simulink model "MSBR_nn_PID_Thot"  (R2016b)
settings: Solver=VariableStepAuto  StartTime=0.0  StopTime=simtime  RelTol=1e-3
values from neighbouring files (symbols this model uses):
  a_b = 1.656E-05    (= 1.656e-05)    [Parameters_new_nodal.m]
  A_Bgn = A_Bg/nn_Bg    [Parameters_new_nodal.m]
  a_f = -8.172E-05    (= -8.172e-05)    [Parameters_new_nodal.m]
  A_fgboren = A_fgbore/nn_fdn    (= 52.5696341877)    [Parameters_new_nodal.m]
  A_fgsleidn = A_fgsleid/nn_fup    (= 29.0039361035)    [Parameters_new_nodal.m]
  A_fgsleodn = A_fgsleod/nn_fdn    (= 43.5059041553)    [Parameters_new_nodal.m]
  a_g = 2.016E-05    (= 2.016e-05)    [Parameters_new_nodal.m]
  A_ggin = A_ggi/nn_gg    [Parameters_new_nodal.m]
  A_ggon = A_ggo/nn_gg    [Parameters_new_nodal.m]
  beta = [2.290E-04, 8.320E-04, 7.100E-04, 8.520E-04, 1.710E-04, 1.020E-04]    [Parameters_new_nodal.m]
  beta_t = sum(beta)    [Parameters_new_nodal.m]
  Cp_B = 9.211E-04    (= 0.0009211)    [Parameters_new_nodal.m]
  Cp_f = 2.302E-03    (= 0.002302)    [Parameters_new_nodal.m]
  Cp_g = 1.679E-03    (= 0.001679)    [Parameters_new_nodal.m]
  h_Bg = 2.839E-03    (= 0.002839)    [Parameters_new_nodal.m]
  h_fgi = 9.176E-03    (= 0.009176)    [Parameters_new_nodal.m]
  h_fgo = 8.165E-03    (= 0.008165)    [Parameters_new_nodal.m]
  h_ggi = cond_g/l_i    [Parameters_new_nodal.m]
  h_ggo = cond_g/l_o    [Parameters_new_nodal.m]
  hA_p1 = h_p*A_phe/4    (= 2.993352)    [Parameters_new_nodal.m]
  hA_p2 = h_p*A_phe/4    (= 2.993352)    [Parameters_new_nodal.m]
  hA_p3 = h_p*A_phe/4    (= 2.993352)    [Parameters_new_nodal.m]
  hA_p4 = h_p*A_phe/4    (= 2.993352)    [Parameters_new_nodal.m]
  hA_pb1 = 7.150E-01    (= 0.715)    [Parameters_new_nodal.m]
  hA_pb2 = 7.150E-01    (= 0.715)    [Parameters_new_nodal.m]
  hA_s1 = h_s*A_phe/4    (= 5.85606)    [Parameters_new_nodal.m]
  hA_s2 = h_s*A_phe/4    (= 5.85606)    [Parameters_new_nodal.m]
  hA_s3 = h_s*A_phe/4    (= 5.85606)    [Parameters_new_nodal.m]
  hA_s4 = h_s*A_phe/4    (= 5.85606)    [Parameters_new_nodal.m]
  hA_s5 = 7.150E-01    (= 0.715)    [Parameters_new_nodal.m]
  hA_s6 = 7.150E-01    (= 0.715)    [Parameters_new_nodal.m]
  k_Ba1 = 8.500E-03/2    (= 0.00425)    [Parameters_new_nodal.m]
  k_Ba2 = 8.500E-03/2    (= 0.00425)    [Parameters_new_nodal.m]
  k_Bb1 = 8.500E-03/2    (= 0.00425)    [Parameters_new_nodal.m]
  k_Bb2 = 8.500E-03/2    (= 0.00425)    [Parameters_new_nodal.m]
  k_BL = 1-k_core    [Parameters_new_nodal.m]
  k_f1a1 = 2.210E-01/2    (= 0.1105)    [Parameters_new_nodal.m]
  k_f1a2 = 2.210E-01/2    (= 0.1105)    [Parameters_new_nodal.m]
  k_f1b1 = 2.210E-01/2    (= 0.1105)    [Parameters_new_nodal.m]
  k_f1b2 = 2.210E-01/2    (= 0.1105)    [Parameters_new_nodal.m]
  k_f2a1 = 2.210E-01/2    (= 0.1105)    [Parameters_new_nodal.m]
  k_f2a2 = 2.210E-01/2    (= 0.1105)    [Parameters_new_nodal.m]
  k_f2b1 = 2.210E-01/2    (= 0.1105)    [Parameters_new_nodal.m]
  k_f2b2 = 2.210E-01/2    (= 0.1105)    [Parameters_new_nodal.m]
  k_g1a = rkmf*m_g1a    [Parameters_new_nodal.m]
  k_g1b = rkmf*m_g1b    [Parameters_new_nodal.m]
  k_g2a = rkmf*m_g2a    [Parameters_new_nodal.m]
  k_g2b = rkmf*m_g2b    [Parameters_new_nodal.m]
  k_g3a = rkmf*m_g3a    [Parameters_new_nodal.m]
  k_g3b = rkmf*m_g3b    [Parameters_new_nodal.m]
  k_g4a = (rkmB*m_gB+rkmf*(m_g4a+m_g4b-m_gB))/2    [Parameters_new_nodal.m]
  k_g4b = (rkmB*m_gB+rkmf*(m_g4a+m_g4b-m_gB))/2    [Parameters_new_nodal.m]
  Lam = 3.300E-04    (= 0.00033)    [Parameters_new_nodal.m]
  lam = [1.260E-02, 3.370E-02, 1.390E-01, 3.250E-01, 1.130E+00, 2.500E+00]    [Parameters_new_nodal.m]
  m_Ba1 = m_B/nn_B    (= 2092.75)    [Parameters_new_nodal.m]
  m_Ba2 = m_B/nn_B    (= 2092.75)    [Parameters_new_nodal.m]
  m_Bb1 = m_B/nn_B    (= 2092.75)    [Parameters_new_nodal.m]
  m_Bb2 = m_B/nn_B    (= 2092.75)    [Parameters_new_nodal.m]
  m_BL = 22804.35    [Parameters_new_nodal.m]
  m_Bm = W_B    (= 271.65)    [Parameters_new_nodal.m]
  m_f1a1 = mn_f    (= 1004.5)    [Parameters_new_nodal.m]
  m_f1a2 = mn_f    (= 1004.5)    [Parameters_new_nodal.m]
  m_f1b1 = mn_f    (= 1004.5)    [Parameters_new_nodal.m]
  m_f1b2 = mn_f    (= 1004.5)    [Parameters_new_nodal.m]
  m_f2a1 = mn_f    (= 1004.5)    [Parameters_new_nodal.m]
  m_f2a2 = mn_f    (= 1004.5)    [Parameters_new_nodal.m]
  m_f2b1 = mn_f    (= 1004.5)    [Parameters_new_nodal.m]
  m_f2b2 = mn_f    (= 1004.5)    [Parameters_new_nodal.m]
  m_g1a = (rho_g*(pi*r_msle^2 - pi*(sle_ID/2)^2)*l_cell*n_cell/2)    [Parameters_new_nodal.m]
  m_g1b = (rho_g*(pi*r_msle^2 - pi*(sle_ID/2)^2)*l_cell*n_cell/2)    [Parameters_new_nodal.m]
  m_g2a = (rho_g*(pi*(sle_OD/2)^2 - pi*r_msle^2)*l_cell*n_cell/2)    [Parameters_new_nodal.m]
  m_g2b = (rho_g*(pi*(sle_OD/2)^2 - pi*r_msle^2)*l_cell*n_cell/2)    [Parameters_new_nodal.m]
  m_g3a = (rho_g*(pi*r_mhex^2 - pi*(bore_OD/2)^2)*l_cell*n_cell/2)    [Parameters_new_nodal.m]
  m_g3b = (rho_g*(pi*r_mhex^2 - pi*(bore_OD/2)^2)*l_cell*n_cell/2)    [Parameters_new_nodal.m]
  m_g4a = (rho_g*(A_hex - pi*r_mhex^2)*l_cell*n_cell/2)    [Parameters_new_nodal.m]
  m_g4b = (rho_g*(A_hex - pi*r_mhex^2)*l_cell*n_cell/2)    [Parameters_new_nodal.m]
  m_pb1 = mcp_pb1/Cp_B    (= 430.680707849)    [Parameters_new_nodal.m]
  m_pb2 = mcp_pb2/Cp_B    (= 430.680707849)    [Parameters_new_nodal.m]
  m_s5 = mcp_s5/Cp_s    (= 1575.26254376)    [Parameters_new_nodal.m]
  m_s6 = mcp_s6/Cp_s    (= 1575.26254376)    [Parameters_new_nodal.m]
  m_sb = 4808    [Parameters_new_nodal.m]
  m_sr = 3062    [Parameters_new_nodal.m]
  mb_cpb = 3.297E+01    (= 32.97)    [Parameters_new_nodal.m]
  mcp_p1 = mn_p*Cp_p    (= 5.3043835)    [Parameters_new_nodal.m]
  mcp_p2 = mn_p*Cp_p    (= 5.3043835)    [Parameters_new_nodal.m]
  mcp_p3 = mn_p*Cp_p    (= 5.3043835)    [Parameters_new_nodal.m]
  mcp_p4 = mn_p*Cp_p    (= 5.3043835)    [Parameters_new_nodal.m]
  mcp_pb1 = 3.967E-01    (= 0.3967)    [Parameters_new_nodal.m]
  mcp_pb2 = 3.967E-01    (= 0.3967)    [Parameters_new_nodal.m]
  mcp_s1 = mn_s*Cp_s    (= 6.80458)    [Parameters_new_nodal.m]
  mcp_s2 = mn_s*Cp_s    (= 6.80458)    [Parameters_new_nodal.m]
  mcp_s3 = mn_s*Cp_s    (= 6.80458)    [Parameters_new_nodal.m]
  mcp_s4 = mn_s*Cp_s    (= 6.80458)    [Parameters_new_nodal.m]
  mcp_s5 = 2.7E+00    (= 2.7)    [Parameters_new_nodal.m]
  mcp_s6 = 2.7E+00    (= 2.7)    [Parameters_new_nodal.m]
  mcp_t1 = 2.158    [Parameters_new_nodal.m]
  mcp_t2 = 2.158    [Parameters_new_nodal.m]
  mcp_t3 = m_t*cp_t    (= 0.51412242)    [Parameters_new_nodal.m]
  mn_m = W_f    (= 1373)    [Parameters_new_nodal.m]
  mn_ms = mn_m    (= 1373)    [Parameters_new_nodal.m]
  mn_p = m_p/nn_p    (= 2304.25)    [Parameters_new_nodal.m]
  mn_s = m_s/nn_s    (= 3970)    [Parameters_new_nodal.m]
  mr_cpr = 1.050E+01    (= 10.5)    [Parameters_new_nodal.m]
  n_frac0 = 1    [Parameters_new_nodal.m]
  P = 556.0    (= 556)    [Parameters_new_nodal.m]
  p_b = 0.87*P    (= 483.72)    [Parameters_new_nodal.m]
  p_r = 0.13*P    (= 72.28)    [Parameters_new_nodal.m]
  T0_b2 = 676.66    [Parameters_new_nodal.m]
  T0_Ba1 = T0_b2-(T0_b2-T_b_in)*(1/4)    (= 662.7725)    [Parameters_new_nodal.m]
  T0_Ba2 = T0_b2    (= 676.66)    [Parameters_new_nodal.m]
  T0_Bb1 = T0_b2-(T0_b2-T_b_in)*(3/4)    (= 634.9975)    [Parameters_new_nodal.m]
  T0_Bb2 = T0_b2-(T0_b2-T_b_in)*(2/4)    (= 648.885)    [Parameters_new_nodal.m]
  T0_BL = T0_Ba2    (= 676.66)    [Parameters_new_nodal.m]
  T0_Bm = T0_Ba2    (= 676.66)    [Parameters_new_nodal.m]
  T0_f1a1 = T0_f4-(T0_f4-Tf_in)*(2/8)    (= 662.7725)    [Parameters_new_nodal.m]
  T0_f1a2 = T0_f4-(T0_f4-Tf_in)*(3/8)    (= 641.93875)    [Parameters_new_nodal.m]
  T0_f1b1 = T0_f4    (= 704.44)    [Parameters_new_nodal.m]
  T0_f1b2 = T0_f4-(T0_f4-Tf_in)*(1/8)    (= 683.60625)    [Parameters_new_nodal.m]
  T0_f2a1 = T0_f4-(T0_f4-Tf_in)*(4/8)    (= 621.105)    [Parameters_new_nodal.m]
  T0_f2a2 = T0_f4-(T0_f4-Tf_in)*(5/8)    (= 600.27125)    [Parameters_new_nodal.m]
  ... (+47 more)
undefined symbols (not defined in the file or in its folder): C0
libraries: simulink x3
settings Model: Creator=VIKRAM SINGH  LastModifiedBy=matthew

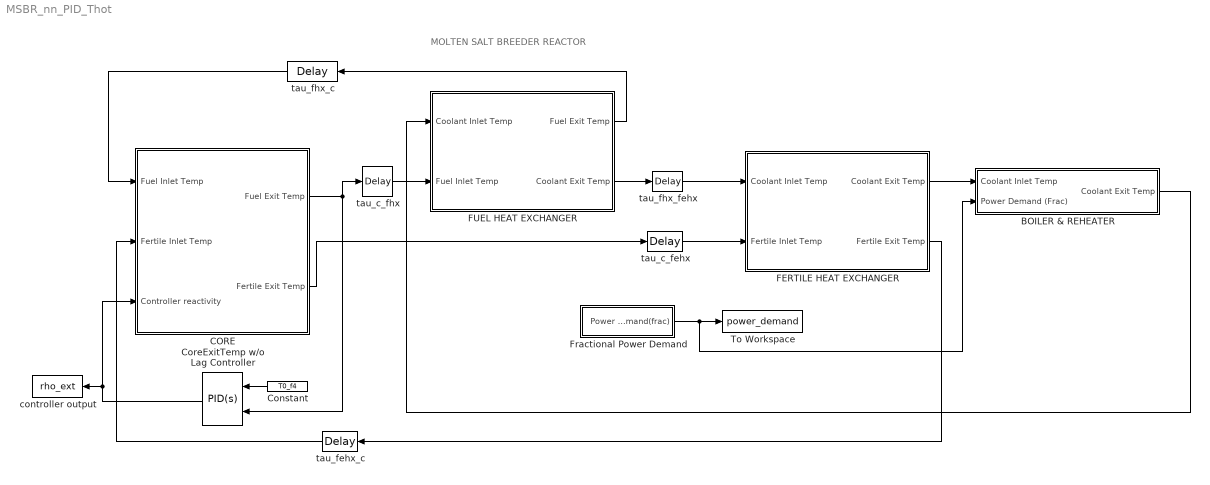
== system MSBR_nn_PID_Thot ==
  note: MOLTEN SALT BREEDER REACTOR
  BOILER & REHEATER : Subsystem
  CORE : Subsystem
  Constant : Constant  Value=T0_f4
  CoreExitTemp w/o Lag Controller : simulink/Continuous/PID Controller (2DOF)  Controller=PID  TimeDomain=Continuous-time  SampleTime=-1  IntegratorMethod=Forward Euler  FilterMethod=Forward Euler  Form=Parallel  UseFilter=on  ControllerParametersSource=internal  P=6.0515509831089e-05  I=4.82645542777223e-05  D=0  N=100  b=1  c=1  InitialConditionSource=internal  InitialConditionForIntegrator=0  InitialConditionForFilter=0  ExternalReset=none  LimitOutput=off  UpperSaturationLimit=inf  LowerSaturationLimit=-inf  LinearizeAsGain=on  AntiWindupMode=none  Kb=1  TrackingMode=off  Kt=1  PParamMin=[]  PParamMax=[]  IParamMin=[]  IParamMax=[]  DParamMin=[]  DParamMax=[]  NParamMin=[]  NParamMax=[]  bParamMin=[]  bParamMax=[]  cParamMin=[]  cParamMax=[]  KbParamMin=[]  KbParamMax=[]  KtParamMin=[]  KtParamMax=[]  POutMin=[]  POutMax=[]  IOutMin=[]  IOutMax=[]  DOutMin=[]  DOutMax=[]  NOutMin=[]  NOutMax=[]  bOutMin=[]  bOutMax=[]  cOutMin=[]  cOutMax=[]  KbOutMin=[]  KbOutMax=[]  KtOutMin=[]  KtOutMax=[]  IntegratorOutMin=[]  IntegratorOutMax=[]  FilterOutMin=[]  FilterOutMax=[]  SumOutMin=[]  SumOutMax=[]  Sum1OutMin=[]  Sum1OutMax=[]  Sum2OutMin=[]  Sum2OutMax=[]  Sum3OutMin=[]  Sum3OutMax=[]  SumI1OutMin=[]  SumI1OutMax=[]  SumI2OutMin=[]  SumI2OutMax=[]  SumI3OutMin=[]  SumI3OutMax=[]  SumDOutMin=[]  SumDOutMax=[]  SaturationOutMin=[]  SaturationOutMax=[]  IntegratorContinuousStateAttributes=''  IntegratorStateMustResolveToSignalObject=off  IntegratorRTWStateStorageClass=Auto  FilterContinuousStateAttributes=''  FilterStateMustResolveToSignalObject=off  FilterRTWStateStorageClass=Auto  DifferentiatorICPrevScaledInput=0  DifferentiatorOutMin=[]  DifferentiatorOutMax=[]
  FERTILE HEAT EXCHANGER : Subsystem
  FUEL HEAT EXCHANGER : Subsystem
  Fractional Power Demand : Subsystem
  To Workspace : ToWorkspace  VariableName=power_demand  SampleTime=-1
  controller output : ToWorkspace  VariableName=rho_ext  SampleTime=-1
  tau_c_fehx : TransportDelay  DelayTime=tau_c_fehx  InitialOutput=T0_b2  BufferSize=4096
  tau_c_fhx : TransportDelay  DelayTime=tau_c_fhx  InitialOutput=T0_f4  BufferSize=4096
  tau_fehx_c : TransportDelay  DelayTime=tau_fehx_c  InitialOutput=T0_pb2  BufferSize=4096
  tau_fhx_c : TransportDelay  DelayTime=tau_fhx_c  InitialOutput=T0_p4  BufferSize=4096
  tau_fhx_fehx : TransportDelay  DelayTime=tau_fhx_fehx  InitialOutput=T0_s4  BufferSize=4096
  wires:
  FUEL HEAT EXCHANGER/2(Coolant Exit Temp) -> tau_fhx_fehx/1
  FERTILE HEAT EXCHANGER/2(Fertile Exit Temp) -> tau_fehx_c/1
  FERTILE HEAT EXCHANGER/1(Coolant Exit Temp) -> BOILER & REHEATER/1(Coolant Inlet Temp)
  tau_c_fhx/1 -> FUEL HEAT EXCHANGER/2(Fuel Inlet Temp)
  tau_c_fehx/1 -> FERTILE HEAT EXCHANGER/2(Fertile Inlet Temp)
  FUEL HEAT EXCHANGER/1(Fuel Exit Temp) -> tau_fhx_c/1
  tau_fhx_fehx/1 -> FERTILE HEAT EXCHANGER/1(Coolant Inlet Temp)
  BOILER & REHEATER/1(Coolant Exit Temp) -> FUEL HEAT EXCHANGER/1(Coolant Inlet Temp)
  tau_fhx_c/1 -> CORE/1(Fuel Inlet Temp)
  tau_fehx_c/1 -> CORE/2(Fertile Inlet Temp)
  CORE/2(Fertile Exit Temp) -> tau_c_fehx/1
  CoreExitTemp w/o Lag Controller/1 -> CORE/3(Controller reactivity), controller output/1
  Fractional Power Demand/1(Power Demand(frac)) -> BOILER & REHEATER/2(Power Demand (Frac)), To Workspace/1
  Constant/1 -> CoreExitTemp w/o Lag Controller/1
  CORE/1(Fuel Exit Temp) -> CoreExitTemp w/o Lag Controller/2, tau_c_fhx/1

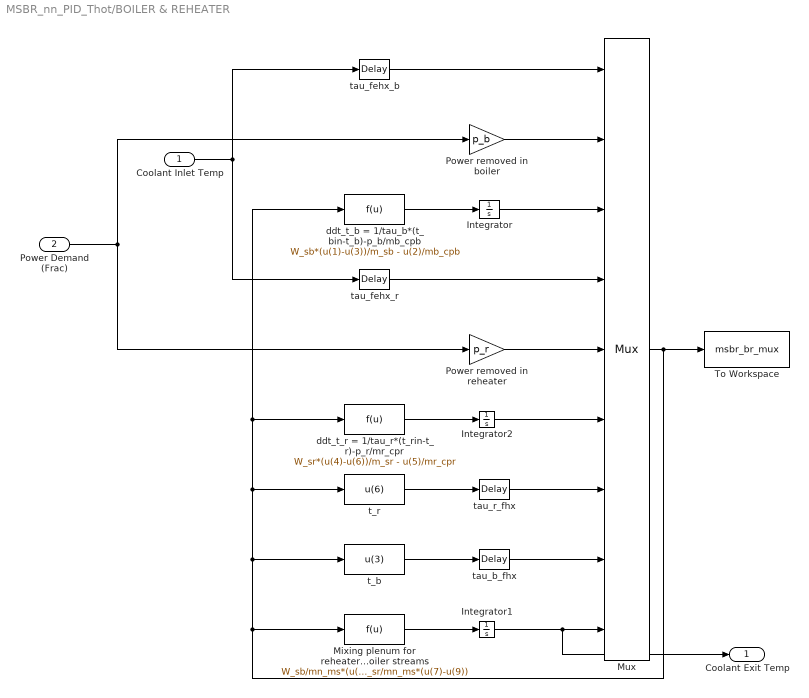
== system MSBR_nn_PID_Thot/BOILER & REHEATER ==
  Coolant Inlet Temp : Inport
  Power Demand (Frac) : Inport  Port=2
  Integrator : Integrator  InitialCondition=Ts_in
  Integrator1 : Integrator  InitialCondition=Ts_in
  Integrator2 : Integrator  InitialCondition=Ts_in
  Mixing plenum for reheater and boiler streams : Fcn  Expr=W_sb/mn_ms*(u(8)-u(9))+W_sr/mn_ms*(u(7)-u(9))
  Mux : Mux  Inputs=9
      settings: DisplayOption=signals
  Power removed in boiler : Gain  Gain=p_b
  Power removed in reheater : Gain  Gain=p_r
  To Workspace : ToWorkspace  VariableName=msbr_br_mux  SampleTime=-1
  ddt_t_b = 1/tau_b*(t_bin-t_b)-p_b/mb_cpb : Fcn  Expr=W_sb*(u(1)-u(3))/m_sb - u(2)/mb_cpb
  ddt_t_r = 1/tau_r*(t_rin-t_r)-p_r/mr_cpr : Fcn  Expr=W_sr*(u(4)-u(6))/m_sr - u(5)/mr_cpr
  t_b : Fcn  Expr=u(3)
  t_r : Fcn  Expr=u(6)
  tau_b_fhx : TransportDelay  DelayTime=tau_b_fhx  InitialOutput=Ts_in  BufferSize=4096
  tau_fehx_b : TransportDelay  DelayTime=tau_fehx_b  InitialOutput=T0_s6  BufferSize=4096
  tau_fehx_r : TransportDelay  DelayTime=tau_fehx_r  InitialOutput=T0_s6  BufferSize=4096
  tau_r_fhx : TransportDelay  DelayTime=tau_r_fhx  InitialOutput=Ts_in  BufferSize=4096
  Coolant Exit Temp : Outport
  wires:
  Coolant Inlet Temp/1 -> tau_fehx_r/1, tau_fehx_b/1
  Power removed in boiler/1 -> Mux/2
  Integrator/1 -> Mux/3
  ddt_t_r = 1/tau_r*(t_rin-t_r)-p_r/mr_cpr/1 -> Integrator2/1
  ddt_t_b = 1/tau_b*(t_bin-t_b)-p_b/mb_cpb/1 -> Integrator/1
  Mux/1 -> t_b/1, t_r/1, ddt_t_r = 1/tau_r*(t_rin-t_r)-p_r/mr_cpr/1, ddt_t_b = 1/tau_b*(t_bin-t_b)-p_b/mb_cpb/1, Mixing plenum for reheater and boiler streams/1, To Workspace/1
  tau_fehx_r/1 -> Mux/4
  Power removed in reheater/1 -> Mux/5
  Integrator2/1 -> Mux/6
  Mixing plenum for reheater and boiler streams/1 -> Integrator1/1
  Integrator1/1 -> Coolant Exit Temp/1, Mux/9
  tau_b_fhx/1 -> Mux/8
  tau_r_fhx/1 -> Mux/7
  t_r/1 -> tau_r_fhx/1
  t_b/1 -> tau_b_fhx/1
  tau_fehx_b/1 -> Mux/1
  Power Demand (Frac)/1 -> Power removed in boiler/1, Power removed in reheater/1

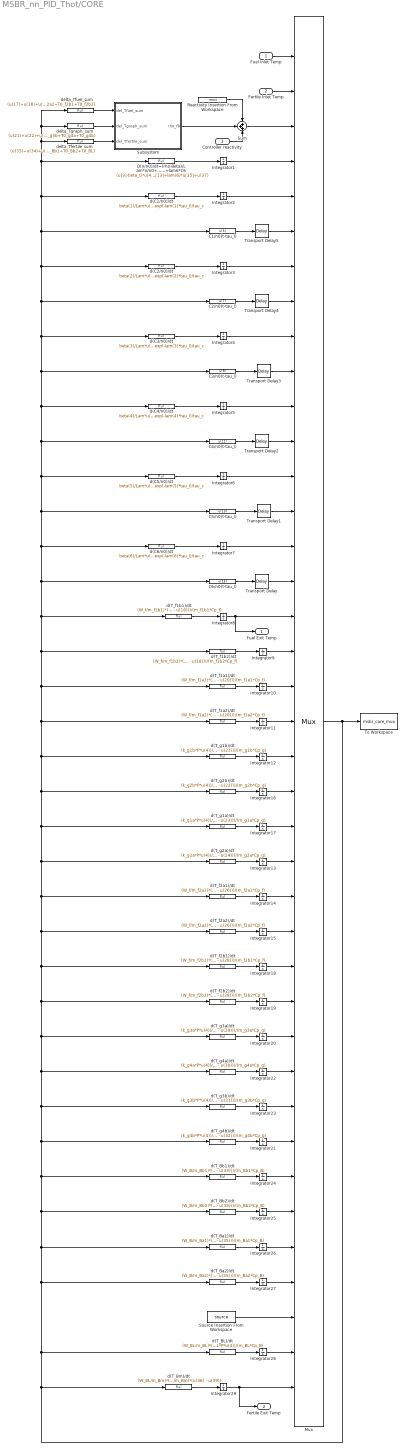
== system MSBR_nn_PID_Thot/CORE ==
  Fuel Inlet Temp : Inport
  Fertile Inlet Temp : Inport  Port=2
  Controller reactivity : Inport  Port=3
  C1/n0(t-tau_l) : Fcn  Expr=u(5)
  C2/n0(t-tau_l) : Fcn  Expr=u(7)
  C3/n0(t-tau_l) : Fcn  Expr=u(9)
  C4/n0(t-tau_l) : Fcn  Expr=u(11)
  C5/n0(t-tau_l) : Fcn  Expr=u(13)
  C6/n0(t-tau_l) : Fcn  Expr=u(15)
  D(n/n0)/dt=(rho-Beta)/Lam*n/n0+lam1*C1+...+lam6*C6 : Fcn  Expr=(u[3]-beta_t)*u[4]/Lam+lam(1)*u[5]+lam(2)*u[7]+lam(3)*u[9]+lam(4)*u[11]+lam(5)*u[13]+lam(6)*u[15]+u(37)
  Integrator1 : Integrator  InitialCondition=n_frac0
  Integrator10 : Integrator  InitialCondition=T0_f1a1
  Integrator11 : Integrator  InitialCondition=T0_f1a2
  Integrator12 : Integrator  InitialCondition=T0_g1b
  Integrator13 : Integrator  InitialCondition=T0_g2a
  Integrator14 : Integrator  InitialCondition=T0_f2a1
  Integrator15 : Integrator  InitialCondition=T0_f2a2
  Integrator16 : Integrator  InitialCondition=T0_g2b
  Integrator17 : Integrator  InitialCondition=T0_g1a
  Integrator18 : Integrator  InitialCondition=T0_f2b1
  Integrator19 : Integrator  InitialCondition=T0_f2b2
  Integrator2 : Integrator  InitialCondition=C0(1)
  Integrator20 : Integrator  InitialCondition=T0_g3a
  Integrator21 : Integrator  InitialCondition=T0_g4b
  Integrator22 : Integrator  InitialCondition=T0_g4a
  Integrator23 : Integrator  InitialCondition=T0_g3b
  Integrator24 : Integrator  InitialCondition=T0_Bb1
  Integrator25 : Integrator  InitialCondition=T0_Bb2
  Integrator26 : Integrator  InitialCondition=T0_Ba1
  Integrator27 : Integrator  InitialCondition=T0_Ba2
  Integrator28 : Integrator  InitialCondition=T0_BL
  Integrator29 : Integrator  InitialCondition=T0_Bm
  Integrator3 : Integrator  InitialCondition=C0(2)
  Integrator4 : Integrator  InitialCondition=C0(3)
  Integrator5 : Integrator  InitialCondition=C0(4)
  Integrator6 : Integrator  InitialCondition=C0(5)
  Integrator7 : Integrator  InitialCondition=C0(6)
  Integrator8 : Integrator  InitialCondition=T0_f1b1
  Integrator9 : Integrator  InitialCondition=T0_f1b2
  Mux : Mux  Inputs=39
      settings: DisplayOption=signals
  Reactivity Insertion From Workspace : FromWorkspace  VariableName=react  SampleTime=1  Interpolate=off  OutputAfterFinalValue=Holding final value
  Source Insertion From Workspace : FromWorkspace  VariableName=source  SampleTime=1  Interpolate=off  OutputAfterFinalValue=Holding final value
  Subsystem : Subsystem
  Sum : Sum  Inputs=+++
  To Workspace : ToWorkspace  VariableName=msbr_core_mux  SampleTime=-1
  Transport Delay : TransportDelay  DelayTime=tau_l  InitialOutput=C0(6)  BufferSize=4096
  Transport Delay1 : TransportDelay  DelayTime=tau_l  InitialOutput=C0(5)  BufferSize=4096
  Transport Delay2 : TransportDelay  DelayTime=tau_l  InitialOutput=C0(4)  BufferSize=4096
  Transport Delay3 : TransportDelay  DelayTime=tau_l  InitialOutput=C0(3)  BufferSize=4096
  Transport Delay4 : TransportDelay  DelayTime=tau_l  InitialOutput=C0(2)  BufferSize=4096
  Transport Delay5 : TransportDelay  DelayTime=tau_l  InitialOutput=C0(1)  BufferSize=4096
  d(C1/n0)/dt : Fcn  Expr=beta(1)/Lam*u(4)-lam(1)*u(5)-u(5)/tau_c+u(6)*exp(-lam(1)*tau_l)/tau_c
  d(C2/n0)/dt : Fcn  Expr=beta(2)/Lam*u(4)-lam(2)*u(7)-u(7)/tau_c+u(8)*exp(-lam(2)*tau_l)/tau_c
  d(C3/n0)/dt : Fcn  Expr=beta(3)/Lam*u(4)-lam(3)*u(9)-u(9)/tau_c+u(10)*exp(-lam(3)*tau_l)/tau_c
  d(C4/n0)/dt : Fcn  Expr=beta(4)/Lam*u(4)-lam(4)*u(11)-u(11)/tau_c+u(12)*exp(-lam(4)*tau_l)/tau_c
  d(C5/n0)/dt : Fcn  Expr=beta(5)/Lam*u(4)-lam(5)*u(13)-u(13)/tau_c+u(14)*exp(-lam(5)*tau_l)/tau_c
  d(C6/n0)/dt : Fcn  Expr=beta(6)/Lam*u(4)-lam(6)*u(15)-u(15)/tau_c+u(16)*exp(-lam(6)*tau_l)/tau_c
  d(T_BL)/dt : Fcn  Expr=(W_BL/m_BL)*(u(2) - u(38)) + (k_BL*P*u(4))/(m_BL*Cp_B)
  d(T_Ba1)/dt : Fcn  Expr=(W_B/m_Ba1)*(u(34) - u(35)) + (k_Ba1*P*u(4))/(m_Ba1*Cp_B) + (h_Bg*A_Bgn*(u(30) - u(35)))/(m_Ba1*Cp_B)
  d(T_Ba2)/dt : Fcn  Expr=(W_B/m_Ba2)*(u(35) - u(36)) + (k_Ba2*P*u(4))/(m_Ba2*Cp_B) + (h_Bg*A_Bgn*(u(30) - u(35)))/(m_Ba2*Cp_B)
  d(T_Bb1)/dt : Fcn  Expr=(W_B/m_Bb1)*(u(2) - u(33)) + (k_Bb1*P*u(4))/(m_Bb1*Cp_B) + (h_Bg*A_Bgn*(u(32) - u(33)))/(m_Bb1*Cp_B)
  d(T_Bb2)/dt : Fcn  Expr=(W_B/m_Bb2)*(u(33) - u(34)) + (k_Bb2*P*u(4))/(m_Bb2*Cp_B) + (h_Bg*A_Bgn*(u(32) - u(33)))/(m_Bb2*Cp_B)
  d(T_Bm)/dt : Fcn  Expr=(W_BL/m_Bm)*(u(38) - u(39)) + (W_B/m_Bm)*(u(36) - u(39))
  d(T_f1a1)/dt : Fcn  Expr=(W_f/m_f1a1)*(u(20) - u(19)) + (k_f1a1*P*u(4))/(m_f1a1*Cp_f) + (h_fgi*A_fgsleidn*(u(23) - u(20)))/(m_f1a1*Cp_f)
  d(T_f1a2)/dt : Fcn  Expr=(W_f/m_f1a2)*(u(25) - u(20)) + (k_f1a2*P*u(4))/(m_f1a2*Cp_f) + (h_fgi*A_fgsleidn*(u(23) - u(20)))/(m_f1a2*Cp_f)
  d(T_f1b1)/dt : Fcn  Expr=(W_f/m_f1b1)*(u(18) - u(17)) + (k_f1b1*P*u(4))/(m_f1b1*Cp_f) + (h_fgi*A_fgsleidn*(u(21) - u(18)))/(m_f1b1*Cp_f)
  d(T_f1b2)/dt : Fcn  Expr=(W_f/m_f1b2)*(u(19) - u(18)) + (k_f1b2*P*u(4))/(m_f1b2*Cp_f) + (h_fgi*A_fgsleidn*(u(21) - u(18)))/(m_f1b2*Cp_f)
  d(T_f2a1)/dt : Fcn  Expr=(W_f/m_f2a1)*(u(26) - u(25)) + (k_f2a1*P*u(4))/(m_f2a1*Cp_f) + (h_fgo*A_fgsleodn*(u(24) - u(26)))/(m_f2a1*Cp_f) + (h_fgo*A_fgboren*(u(29) - u(26)))/(m_f2a1*Cp_f)
  d(T_f2a2)/dt : Fcn  Expr=(W_f/m_f2a2)*(u(27) - u(26)) + (k_f2a2*P*u(4))/(m_f2a2*Cp_f) + (h_fgo*A_fgsleodn*(u(24) - u(26)))/(m_f2a2*Cp_f) + (h_fgo*A_fgboren*(u(29) - u(26)))/(m_f2a2*Cp_f)
  d(T_f2b1)/dt : Fcn  Expr=(W_f/m_f2b1)*(u(28) - u(27)) + (k_f2b1*P*u(4))/(m_f2b1*Cp_f) + (h_fgo*A_fgsleodn*(u(22) - u(28)))/(m_f2b1*Cp_f) + (h_fgo*A_fgboren*(u(31) - u(28)))/(m_f2b1*Cp_f)
  d(T_f2b2)/dt : Fcn  Expr=(W_f/m_f2b2)*(u(1) - u(28)) + (k_f2b2*P*u(4))/(m_f2b2*Cp_f) + (h_fgo*A_fgsleodn*(u(22) - u(28)))/(m_f2b2*Cp_f) + (h_fgo*A_fgboren*(u(31) - u(28)))/(m_f2b2*Cp_f)
  d(T_g1a)/dt : Fcn  Expr=(k_g1a*P*u(4))/(m_g1a*Cp_g) + (2*h_fgi*A_fgsleidn*(u(20) - u(23)))/(m_g1a*Cp_g) + (h_ggi*A_ggin*(u(24) - u(23)))/(m_g1a*Cp_g)
  d(T_g1b)/dt : Fcn  Expr=(k_g1b*P*u(4))/(m_g1b*Cp_g) + (2*h_fgi*A_fgsleidn*(u(18) - u(21)))/(m_g1b*Cp_g) + (h_ggi*A_ggin*(u(22) - u(21)))/(m_g1b*Cp_g)
  d(T_g2a)/dt : Fcn  Expr=(k_g2a*P*u(4))/(m_g2a*Cp_g) + (2*h_fgo*A_fgsleodn*(u(26) - u(24)))/(m_g2a*Cp_g) + (h_ggi*A_ggin*(u(23) - u(24)))/(m_g2a*Cp_g)
  d(T_g2b)/dt : Fcn  Expr=(k_g2b*P*u(4))/(m_g2b*Cp_g) + (2*h_fgo*A_fgsleodn*(u(28) - u(22)))/(m_g2b*Cp_g) + (h_ggi*A_ggin*(u(21) - u(22)))/(m_g2b*Cp_g)
  d(T_g3a)/dt : Fcn  Expr=(k_g3a*P*u(4))/(m_g3a*Cp_g) + (2*h_fgo*A_fgboren*(u(26) - u(29)))/(m_g3a*Cp_g) + (h_ggo*A_ggon*(u(30) - u(29)))/(m_g3a*Cp_g)
  d(T_g3b)/dt : Fcn  Expr=(k_g3b*P*u(4))/(m_g3b*Cp_g) + (2*h_fgo*A_fgboren*(u(28) - u(31)))/(m_g3b*Cp_g) + (h_ggo*A_ggon*(u(32) - u(31)))/(m_g3b*Cp_g)
  d(T_g4a)/dt : Fcn  Expr=(k_g4a*P*u(4))/(m_g4a*Cp_g) + (2*h_Bg*A_Bgn*(u(35) - u(30)))/(m_g4a*Cp_g) + (h_ggo*A_ggon*(u(29) - u(30)))/(m_g4a*Cp_g)
  d(T_g4b)/dt : Fcn  Expr=(k_g4b*P*u(4))/(m_g4b*Cp_g) + (2*h_Bg*A_Bgn*(u(33) - u(32)))/(m_g4b*Cp_g) + (h_ggo*A_ggon*(u(31) - u(32)))/(m_g4b*Cp_g)
  delta_Tfertile_sum : Fcn  Expr=(u(33)+u(34)+u(35)+u(36)+u(38)) - (T0_Ba1+T0_Ba2+T0_Bb1+T0_Bb2+T0_BL)
  delta_Tfuel_sum : Fcn  Expr=(u(17)+u(18)+u(19)+u(20)+u(25)+u(26)+u(27)+u(28)) - (T0_f1a1+T0_f1a2+T0_f1b1+T0_f1b2+T0_f2a1+T0_f2a2+T0_f2b1+T0_f2b2)
  delta_Tgraph_sum : Fcn  Expr=(u(21)+u(22)+u(23)+u(24)+u(29)+u(30)+u(31)+u(32)) - (T0_g1a+T0_g1b+T0_g2a+T0_g2b+T0_g3a+T0_g3b+T0_g4a+T0_g4b)
  Fuel Exit Temp : Outport
  Fertile Exit Temp : Outport  Port=2
  wires:
  d(T_f1b1)/dt/1 -> Integrator8/1
  d(T_f1b2)/dt/1 -> Integrator9/1
  d(T_f1a1)/dt/1 -> Integrator10/1
  d(T_f1a2)/dt/1 -> Integrator11/1
  d(T_g1b)/dt/1 -> Integrator12/1
  Integrator12/1 -> Mux/21
  Integrator11/1 -> Mux/20
  Integrator10/1 -> Mux/19
  Integrator9/1 -> Mux/18
  Integrator8/1 -> Fuel Exit Temp/1, Mux/17
  D(n/n0)/dt=(rho-Beta)/Lam*n/n0+lam1*C1+...+lam6*C6/1 -> Integrator1/1
  d(C1/n0)/dt/1 -> Integrator2/1
  d(C2/n0)/dt/1 -> Integrator3/1
  d(C3/n0)/dt/1 -> Integrator4/1
  d(C4/n0)/dt/1 -> Integrator5/1
  d(C5/n0)/dt/1 -> Integrator6/1
  d(C6/n0)/dt/1 -> Integrator7/1
  C6/n0(t-tau_l)/1 -> Transport Delay/1
  Transport Delay/1 -> Mux/16
  C5/n0(t-tau_l)/1 -> Transport Delay1/1
  Transport Delay1/1 -> Mux/14
  Transport Delay2/1 -> Mux/12
  C4/n0(t-tau_l)/1 -> Transport Delay2/1
  C3/n0(t-tau_l)/1 -> Transport Delay3/1
  Transport Delay3/1 -> Mux/10
  Transport Delay4/1 -> Mux/8
  C2/n0(t-tau_l)/1 -> Transport Delay4/1
  Transport Delay5/1 -> Mux/6
  C1/n0(t-tau_l)/1 -> Transport Delay5/1
  Sum/1 -> Mux/3
  delta_Tfuel_sum/1 -> Subsystem/1(del_Tfuel_sum)
  delta_Tgraph_sum/1 -> Subsystem/2(del_Tgraph_sum)
  delta_Tfertile_sum/1 -> Subsystem/3(del_Tfertile_sum)
  Source Insertion From Workspace/1 -> Mux/37
  d(T_g2b)/dt/1 -> Integrator16/1
  d(T_g1a)/dt/1 -> Integrator17/1
  d(T_g2a)/dt/1 -> Integrator13/1
  d(T_f2a1)/dt/1 -> Integrator14/1
  d(T_f2a2)/dt/1 -> Integrator15/1
  Integrator15/1 -> Mux/26
  Integrator14/1 -> Mux/25
  Integrator13/1 -> Mux/24
  Integrator17/1 -> Mux/23
  Integrator16/1 -> Mux/22
  d(T_f2b1)/dt/1 -> Integrator18/1
  d(T_f2b2)/dt/1 -> Integrator19/1
  Integrator18/1 -> Mux/27
  d(T_g3a)/dt/1 -> Integrator20/1
  Integrator20/1 -> Mux/29
  d(T_g4a)/dt/1 -> Integrator22/1
  d(T_g3b)/dt/1 -> Integrator23/1
  d(T_g4b)/dt/1 -> Integrator21/1
  Integrator21/1 -> Mux/32
  Integrator23/1 -> Mux/31
  Integrator22/1 -> Mux/30
  d(T_Bb1)/dt/1 -> Integrator24/1
  d(T_Bb2)/dt/1 -> Integrator25/1
  Integrator25/1 -> Mux/34
  Integrator24/1 -> Mux/33
  d(T_Ba1)/dt/1 -> Integrator26/1
  d(T_Ba2)/dt/1 -> Integrator27/1
  Integrator27/1 -> Mux/36
  Integrator26/1 -> Mux/35
  Mux/1 -> d(T_Bm)/dt/1, d(T_BL)/dt/1, d(T_Ba2)/dt/1, d(T_Ba1)/dt/1, d(T_Bb2)/dt/1, d(T_Bb1)/dt/1, d(T_g4b)/dt/1, d(T_g3b)/dt/1, d(T_g4a)/dt/1, d(T_g3a)/dt/1, d(T_f2b2)/dt/1, d(T_f2b1)/dt/1, d(T_f2a2)/dt/1, d(T_f2a1)/dt/1, d(T_g2a)/dt/1, d(T_g1a)/dt/1, d(T_g2b)/dt/1, delta_Tfertile_sum/1, delta_Tgraph_sum/1, delta_Tfuel_sum/1, D(n/n0)/dt=(rho-Beta)/Lam*n/n0+lam1*C1+...+lam6*C6/1, d(C1/n0)/dt/1, C1/n0(t-tau_l)/1, d(C2/n0)/dt/1, C2/n0(t-tau_l)/1, d(C3/n0)/dt/1, C3/n0(t-tau_l)/1, d(C4/n0)/dt/1, C4/n0(t-tau_l)/1, d(C5/n0)/dt/1, C5/n0(t-tau_l)/1, d(C6/n0)/dt/1, C6/n0(t-tau_l)/1, d(T_f1b1)/dt/1, d(T_f1b2)/dt/1, d(T_f1a1)/dt/1, d(T_f1a2)/dt/1, d(T_g1b)/dt/1, To Workspace/1
  Integrator19/1 -> Mux/28
  d(T_BL)/dt/1 -> Integrator28/1
  Integrator28/1 -> Mux/38
  d(T_Bm)/dt/1 -> Integrator29/1
  Integrator29/1 -> Fertile Exit Temp/1, Mux/39
  Fertile Inlet Temp/1 -> Mux/2
  Fuel Inlet Temp/1 -> Mux/1
  Controller reactivity/1 -> Sum/3
  Subsystem/1(rho_fb) -> Sum/2
  Integrator1/1 -> Mux/4
  Integrator2/1 -> Mux/5
  Integrator3/1 -> Mux/7
  Integrator4/1 -> Mux/9
  Integrator5/1 -> Mux/11
  Integrator6/1 -> Mux/13
  Integrator7/1 -> Mux/15
  Reactivity Insertion From Workspace/1 -> Sum/1

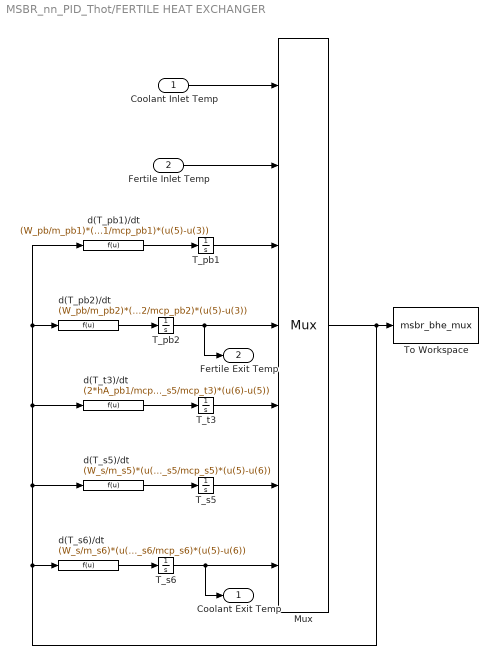
== system MSBR_nn_PID_Thot/FERTILE HEAT EXCHANGER ==
  Coolant Inlet Temp : Inport
  Fertile Inlet Temp : Inport  Port=2
  Mux : Mux  Inputs=7
      settings: DisplayOption=signals
  T_pb1 : Integrator  InitialCondition=T0_pb1
  T_pb2 : Integrator  InitialCondition=T0_pb2
  "T_s5 " : Integrator  InitialCondition=T0_s5
  T_s6 : Integrator  InitialCondition=T0_s6
  T_t3 : Integrator  InitialCondition=T0_t3
  To Workspace : ToWorkspace  VariableName=msbr_bhe_mux  SampleTime=-1
  d(T_pb1)/dt : Fcn  Expr=(W_pb/m_pb1)*(u(2)-u(3)) + (hA_pb1/mcp_pb1)*(u(5)-u(3))
  d(T_pb2)/dt : Fcn  Expr=(W_pb/m_pb2)*(u(3)-u(4)) + (hA_pb2/mcp_pb2)*(u(5)-u(3))
  d(T_s5)/dt : Fcn  Expr=(W_s/m_s5)*(u(1)-u(6))+(hA_s5/mcp_s5)*(u(5)-u(6))
  d(T_s6)/dt : Fcn  Expr=(W_s/m_s6)*(u(6)-u(7))+(hA_s6/mcp_s6)*(u(5)-u(6))
  d(T_t3)/dt : Fcn  Expr=(2*hA_pb1/mcp_t3)*(u(3)-u(5)) + (2*hA_s5/mcp_t3)*(u(6)-u(5))
  Coolant Exit Temp : Outport
  Fertile Exit Temp : Outport  Port=2
  wires:
  d(T_pb1)/dt/1 -> T_pb1/1
  d(T_pb2)/dt/1 -> T_pb2/1
  d(T_t3)/dt/1 -> T_t3/1
  d(T_s5)/dt/1 -> "T_s5 "/1
  d(T_s6)/dt/1 -> T_s6/1
  T_s6/1 -> Mux/7, Coolant Exit Temp/1
  "T_s5 "/1 -> Mux/6
  T_t3/1 -> Mux/5
  T_pb2/1 -> Fertile Exit Temp/1, Mux/4
  T_pb1/1 -> Mux/3
  Mux/1 -> d(T_s6)/dt/1, d(T_s5)/dt/1, d(T_t3)/dt/1, d(T_pb2)/dt/1, d(T_pb1)/dt/1, To Workspace/1
  Coolant Inlet Temp/1 -> Mux/1
  Fertile Inlet Temp/1 -> Mux/2

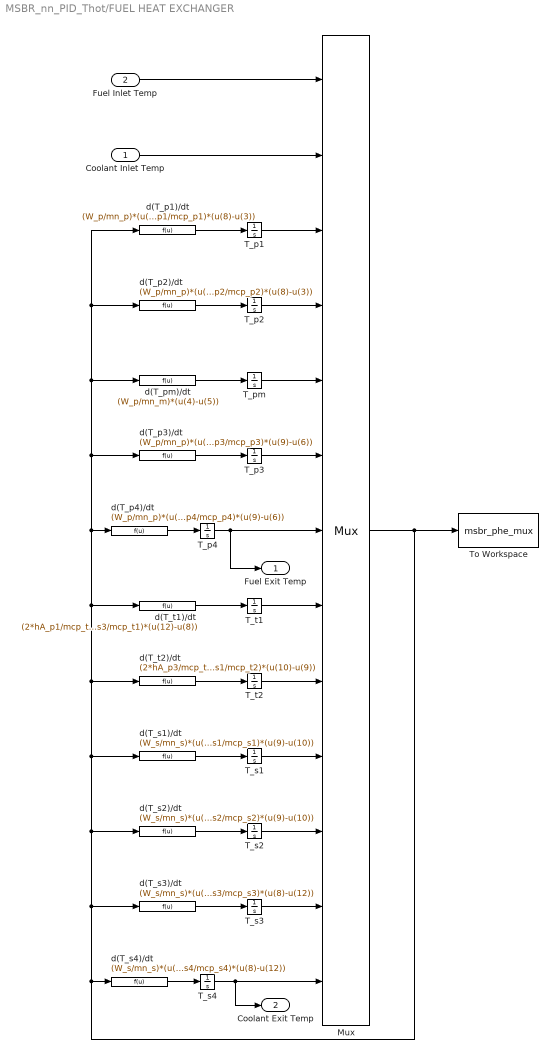
== system MSBR_nn_PID_Thot/FUEL HEAT EXCHANGER ==
  Coolant Inlet Temp : Inport
  Fuel Inlet Temp : Inport  Port=2
  Mux : Mux  Inputs=13
      settings: DisplayOption=signals
  T_p1 : Integrator  InitialCondition=T0_p1
  T_p2 : Integrator  InitialCondition=T0_p2
  "T_p3 " : Integrator  InitialCondition=T0_p3
  T_p4 : Integrator  InitialCondition=T0_p4
  T_pm : Integrator  InitialCondition=T0_pm
  T_s1 : Integrator  InitialCondition=T0_s1
  T_s2 : Integrator  InitialCondition=T0_s2
  T_s3 : Integrator  InitialCondition=T0_s3
  T_s4 : Integrator  InitialCondition=T0_s4
  T_t1 : Integrator  InitialCondition=T0_t1
  T_t2 : Integrator  InitialCondition=T0_t2
  To Workspace : ToWorkspace  VariableName=msbr_phe_mux  SampleTime=-1
  d(T_p1)/dt : Fcn  Expr=(W_p/mn_p)*(u(1)-u(3)) + (hA_p1/mcp_p1)*(u(8)-u(3))
  d(T_p2)/dt : Fcn  Expr=(W_p/mn_p)*(u(3)-u(4)) + (hA_p2/mcp_p2)*(u(8)-u(3))
  d(T_p3)/dt : Fcn  Expr=(W_p/mn_p)*(u(5)-u(6)) + (hA_p3/mcp_p3)*(u(9)-u(6))
  d(T_p4)/dt : Fcn  Expr=(W_p/mn_p)*(u(6)-u(7)) + (hA_p4/mcp_p4)*(u(9)-u(6))
  d(T_pm)/dt : Fcn  Expr=(W_p/mn_m)*(u(4)-u(5))
  d(T_s1)/dt : Fcn  Expr=(W_s/mn_s)*(u(2)-u(10)) + (hA_s1/mcp_s1)*(u(9)-u(10))
  d(T_s2)/dt : Fcn  Expr=(W_s/mn_s)*(u(10)-u(11)) + (hA_s2/mcp_s2)*(u(9)-u(10))
  d(T_s3)/dt : Fcn  Expr=(W_s/mn_s)*(u(11)-u(12)) + (hA_s3/mcp_s3)*(u(8)-u(12))
  d(T_s4)/dt : Fcn  Expr=(W_s/mn_s)*(u(12)-u(13)) + (hA_s4/mcp_s4)*(u(8)-u(12))
  d(T_t1)/dt : Fcn  Expr=(2*hA_p1/mcp_t1)*(u(3)-u(8)) + (2*hA_s3/mcp_t1)*(u(12)-u(8))
  d(T_t2)/dt : Fcn  Expr=(2*hA_p3/mcp_t2)*(u(6)-u(9)) + (2*hA_s1/mcp_t2)*(u(10)-u(9))
  Fuel Exit Temp : Outport
  Coolant Exit Temp : Outport  Port=2
  wires:
  Fuel Inlet Temp/1 -> Mux/1
  Coolant Inlet Temp/1 -> Mux/2
  d(T_p1)/dt/1 -> T_p1/1
  d(T_p2)/dt/1 -> T_p2/1
  d(T_pm)/dt/1 -> T_pm/1
  d(T_p3)/dt/1 -> "T_p3 "/1
  d(T_p4)/dt/1 -> T_p4/1
  d(T_t1)/dt/1 -> T_t1/1
  d(T_t2)/dt/1 -> T_t2/1
  d(T_s1)/dt/1 -> T_s1/1
  d(T_s2)/dt/1 -> T_s2/1
  T_s2/1 -> Mux/11
  T_s1/1 -> Mux/10
  T_t2/1 -> Mux/9
  T_t1/1 -> Mux/8
  T_p4/1 -> Mux/7, Fuel Exit Temp/1
  "T_p3 "/1 -> Mux/6
  T_pm/1 -> Mux/5
  T_p2/1 -> Mux/4
  T_p1/1 -> Mux/3
  d(T_s3)/dt/1 -> T_s3/1
  d(T_s4)/dt/1 -> T_s4/1
  T_s4/1 -> Coolant Exit Temp/1, Mux/13
  T_s3/1 -> Mux/12
  Mux/1 -> d(T_s4)/dt/1, d(T_s3)/dt/1, d(T_s2)/dt/1, d(T_s1)/dt/1, d(T_t2)/dt/1, d(T_t1)/dt/1, d(T_p4)/dt/1, d(T_p3)/dt/1, d(T_pm)/dt/1, d(T_p2)/dt/1, d(T_p1)/dt/1, To Workspace/1

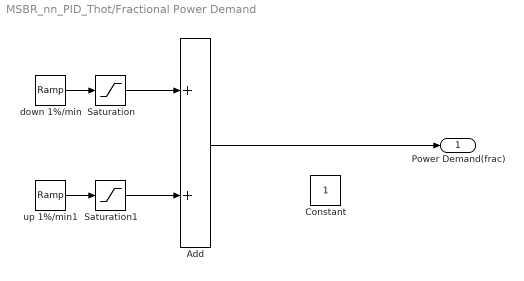
== system MSBR_nn_PID_Thot/Fractional Power Demand ==
  Add : Sum
  Constant : Constant
  Saturation : Saturate  UpperLimit=1  LowerLimit=0.5
  Saturation1 : Saturate  LowerLimit=0
  down 1%/min : simulink/Sources/Ramp  slope=-0.01/60  start=2000  X0=1
  up 1%/min1 : simulink/Sources/Ramp  slope=0.01/60  start=3000+5000  X0=0
  Power Demand(frac) : Outport
  wires:
  down 1%/min/1 -> Saturation/1
  Saturation/1 -> Add/1
  up 1%/min1/1 -> Saturation1/1
  Saturation1/1 -> Add/2
  Add/1 -> Power Demand(frac)/1

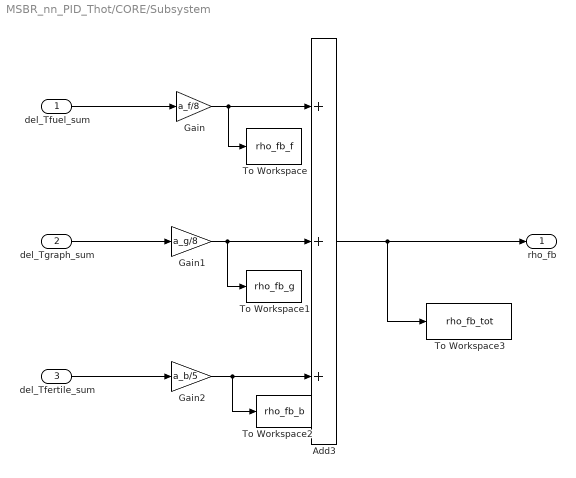
== system MSBR_nn_PID_Thot/CORE/Subsystem ==
  del_Tfuel_sum : Inport
  del_Tgraph_sum : Inport  Port=2
  del_Tfertile_sum : Inport  Port=3
  Add3 : Sum  Inputs=+++
  Gain : Gain  Gain=a_f/8
  Gain1 : Gain  Gain=a_g/8
  Gain2 : Gain  Gain=a_b/5
  To Workspace : ToWorkspace  VariableName=rho_fb_f  SampleTime=-1
  To Workspace1 : ToWorkspace  VariableName=rho_fb_g  SampleTime=-1
  To Workspace2 : ToWorkspace  VariableName=rho_fb_b  SampleTime=-1
  To Workspace3 : ToWorkspace  VariableName=rho_fb_tot  SampleTime=-1
  rho_fb : Outport
  wires:
  del_Tfuel_sum/1 -> Gain/1
  del_Tgraph_sum/1 -> Gain1/1
  del_Tfertile_sum/1 -> Gain2/1
  Gain1/1 -> To Workspace1/1, Add3/2
  Gain/1 -> To Workspace/1, Add3/1
  Add3/1 -> To Workspace3/1, rho_fb/1
  Gain2/1 -> To Workspace2/1, Add3/3
